simulink model "rotpentemplate"  (R2020b)
settings: Solver=ode45  StartTime=0.0  StopTime=30  RelTol=1e-3  EnableMultiTasking=on
values from neighbouring files (symbols this model uses):
  adingain = [adingain 1 1 1 1 1]    [hwinit.m]
  adinoffs = [adinoffs 0 0 0 0 0]    [hwinit.m]
  daoutgain = 1*[-6]    [hwinit.m]
  daoutoffs = -[-0.0025]    [hwinit.m]
undefined symbols (not defined in the file or in its folder): Discrete, h, Kd, Ld, R, sysd, Time
libraries: simulink x5, sharedTrackingLibrary x1, ctrlSharedLib x1
settings Model: Creator=rbabuska  LastModifiedBy=fballast
settings DataIOCC: LimitDataPoints=on  SaveFormat=Array  ReturnWorkspaceOutputs=off  SignalLoggingName=sigsOut
settings OptimizationCC: BooleanDataType=off  ExpressionDepthLimit=2147483647  InitFltsAndDblsToZero=on  LifeSpan=inf
settings DebuggingCC: SaveWithParameterizedLinksMsg=none  SignalResolutionControl=TryResolveAllWithWarning  MultiTaskDSMMsg=warning  MultiTaskCondExecSysMsg=none  AllowSymbolicDim=off  StateNameClashWarn=warning  SFUnexpectedBacktrackingDiag=warning  SFNoUnconditionalDefaultTransitionDiag=warning  SFExecutionAtInitializationDiag=none  ArithmeticOperatorsInVariantConditions=warning
settings HardwareCC: ProdBitPerPointer=32  ProdBitPerSizeT=32  ProdBitPerPtrDiffT=32  ProdLargestAtomicFloat=None  ProdIntDivRoundTo=Undefined  ProdEndianess=Unspecified  ProdWordSize=32  ProdHWDeviceType=32-bit Generic  TargetUnknown=on
settings ModelReferenceCC: PropagateSignalLabelsOutOfModel=off
settings SFSimCC: SimUseLocalCustomCode=off  CustomCodeUndefinedFunction=UseInterfaceOnly
settings RTWCC: RTWUseLocalCustomCode=off
settings CodeAppCC: StateflowObjectComments=on
settings GRTTargetCC: TargetFcnLib=ansi_tfl_tmw.mat  TargetLangStandard=C89/C90 (ANSI)  CombineOutputUpdateFcns=off  GRTInterface=on
settings ConfigComp: CovMetricSettings=dw  CovSaveCumulativeToWorkspaceVar=on  CovSaveSingleToWorkspaceVar=on  CovExternalEMLEnable=off

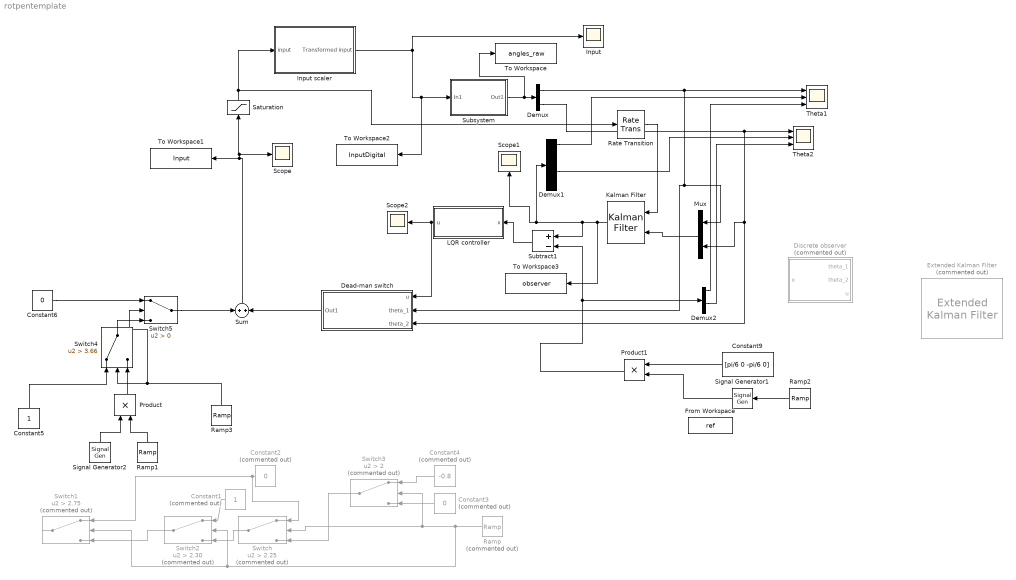
== system rotpentemplate ==
  Constant1 : Constant  Commented=on
  Constant2 : Constant  Commented=on  Value=0
  Constant3 : Constant  Commented=on  Value=0
  Constant4 : Constant  Commented=on  Value=-0.8
  Constant5 : Constant
  Constant6 : Constant  Value=0
  Constant9 : Constant  Value=[pi/6 0 -pi/6 0]
  Dead-man switch : Subsystem
  Demux : Demux  Outputs=2
  Demux1 : Demux
  Demux2 : Demux
  Discrete observer : Subsystem  Commented=on
  Extended Kalman Filter : sharedTrackingLibrary/Extended Kalman Filter  Commented=on  StateTransitionFcn=nonlin_state  HasStateTransitionJacobianFcn=off  HasAdditiveProcessNoise=Additive  ProcessNoise=Q  HasTimeVaryingProcessNoise=off  HasStateTransitionFcnExtraArgument=1  InitialState=[0;0;0;0]  InitialStateCovariance=1.0e-1  MeasurementFcn1=nonlin_meas  HasMeasurementJacobianFcn1=off  HasMeasurementEnablePort1=off  HasAdditiveMeasurementNoise1=Additive  MeasurementNoise1=R  HasTimeVaryingMeasurementNoise1=off  HasMeasurementFcnExtraArgument1=0  MeasurementFcn2=myMeasurementFcn  HasMeasurementJacobianFcn2=off  HasMeasurementEnablePort2=off  HasAdditiveMeasurementNoise2=Additive  MeasurementNoise2=1  HasTimeVaryingMeasurementNoise2=off  HasMeasurementFcnExtraArgument2=0  MeasurementFcn3=myMeasurementFcn  HasMeasurementJacobianFcn3=off  HasMeasurementEnablePort3=off  HasAdditiveMeasurementNoise3=Additive  MeasurementNoise3=1  HasTimeVaryingMeasurementNoise3=off  HasMeasurementFcnExtraArgument3=0  MeasurementFcn4=myMeasurementFcn  HasMeasurementJacobianFcn4=off  HasMeasurementEnablePort4=off  HasAdditiveMeasurementNoise4=Additive  MeasurementNoise4=1  HasTimeVaryingMeasurementNoise4=off  HasMeasurementFcnExtraArgument4=0  MeasurementFcn5=myMeasurementFcn  HasMeasurementJacobianFcn5=off  HasMeasurementEnablePort5=off  HasAdditiveMeasurementNoise5=Additive  MeasurementNoise5=1  HasTimeVaryingMeasurementNoise5=off  HasMeasurementFcnExtraArgument5=0  EnableMultirate=off  StateTransitionFcnSampleTime=1  MeasurementFcn1SampleTime=1  MeasurementFcn2SampleTime=1  MeasurementFcn3SampleTime=1  MeasurementFcn4SampleTime=1  MeasurementFcn5SampleTime=1  UseCurrentEstimator=on  OutputStateCovariance=off  DataType=double  SampleTime=0.01  NumberOfMeasurements=1
      settings: SourceProductBaseCode=CT,DR,TF,ID,LP,NV,AR,RO,RR,UV,VE
  From Workspace : FromWorkspace  VariableName=ref
  Input : Scope
  Input scaler : Subsystem
  Kalman Filter : ctrlSharedLib/Kalman Filter  TimeDomain=Discrete-Time  UseCurrentEstimator=on  ModelSource=LTI State-Space Variable  ModelSourceVariable=sysd  A=0.95  B=1  C=1  D=0  NumberOfStates=1  NumberOfInputs=1  NumberOfOutputs=1  InitialEstimateSource=Dialog  X0=0  P0=10  UseK=off  UseGH=off  NumberOfProcessNoiseInputs=1  G=eye(4)  TimeInvariantG=on  H=0  TimeInvariantH=on  Q=Q  TimeInvariantQ=on  R=R  TimeInvariantR=on  N=0  TimeInvariantN=on  AddInputPort=on  AddEnablePort=off  OutputEstimatedY=off  OutputP=off  Ts=-1
  LQR controller : Subsystem
  Mux : Mux  Inputs=2
  Product : Product
  Product1 : Product
  Ramp : simulink/Sources/Ramp  Commented=on  slope=1  start=0  InitialOutput=0
  Ramp1 : simulink/Sources/Ramp  slope=0.76  start=0.86  InitialOutput=0
  Ramp2 : simulink/Sources/Ramp  slope=1  start=3  InitialOutput=0
  Ramp3 : simulink/Sources/Ramp  slope=1  start=0  InitialOutput=0
  Rate Transition : RateTransition  OutPortSampleTime=h
  Saturation : Saturate  UpperLimit=1  LowerLimit=-1
  Scope : Scope
  Scope1 : Scope
  Scope2 : Scope
  Signal Generator1 : SignalGenerator  TimeSource=Use external signal  Amplitude=0  Frequency=0.1
  Signal Generator2 : SignalGenerator  Frequency=1.15
  Subsystem : Subsystem
      mask Display: disp('Rotational\nPendulum')
  Subtract1 : Sum  Inputs=+-
  Sum : Sum  Inputs=+|+
  Switch : Switch  Commented=on  Criteria=u2 > Threshold  Threshold=2.25
  Switch1 : Switch  Commented=on  Criteria=u2 > Threshold  Threshold=2.75
  Switch2 : Switch  Commented=on  Criteria=u2 > Threshold  Threshold=2.30
  Switch3 : Switch  Commented=on  Criteria=u2 > Threshold  Threshold=2
  Switch4 : Switch  Criteria=u2 > Threshold  Threshold=3.66
  Switch5 : Switch  Criteria=u2 > Threshold
  Theta1 : Scope  NumInputPorts=3
  Theta2 : Scope  NumInputPorts=3
  To Workspace : ToWorkspace  VariableName=angles_raw  SaveFormat=Timeseries  SampleTime=-1
  To Workspace1 : ToWorkspace  VariableName=Input  SaveFormat=Timeseries  SampleTime=-1
  To Workspace2 : ToWorkspace  VariableName=InputDigital  SaveFormat=Timeseries  SampleTime=-1
  To Workspace3 : ToWorkspace  VariableName=observer  SaveFormat=Timeseries  SampleTime=-1
  wires:
  Input scaler/1(Transformed input) -> To Workspace2/1, Subsystem/1(In1), Input/1
  Subsystem/1(Out1) -> To Workspace/1, Demux/1
  Demux/1 -> Theta1/1, Dead-man switch/2(theta_1), Mux/1
  Kalman Filter/1 -> To Workspace3/1, Subtract1/1, Scope1/1, Demux1/1
  Demux/2 -> Dead-man switch/3(theta_2), Mux/2, Theta2/1
  LQR controller/1(u) -> Scope2/1, Dead-man switch/1(u)
  Demux1/1 -> Theta1/2
  Demux1/3 -> Theta2/2
  Mux/1 -> Kalman Filter/2
  Rate Transition/1 -> Kalman Filter/1
  Subtract1/1 -> LQR controller/1(x)
  Demux2/1 -> Theta1/3
  Demux2/3 -> Theta2/3
  Ramp2/1 -> Signal Generator1/1
  Constant9/1 -> Product1/1
  Sum/1 -> To Workspace1/1, Scope/1, Saturation/1
  Switch3/1 -> Switch/3
  Ramp/1 -> Switch3/2, Switch/2, Switch2/2, Switch1/2
  Switch2/1 -> Switch1/3
  Constant2/1 -> Switch/1, Switch1/1
  Dead-man switch/1(Out1) -> Sum/2
  Constant1/1 -> Switch2/1
  Switch/1 -> Switch2/3
  Constant3/1 -> Switch3/3
  Constant4/1 -> Switch3/1
  Signal Generator2/1 -> Product/1
  Ramp1/1 -> Product/2
  Product/1 -> Switch4/3
  Constant5/1 -> Switch4/1
  Ramp3/1 -> Switch5/2, Switch4/2
  Switch5/1 -> Sum/1
  Constant6/1 -> Switch5/1
  Switch4/1 -> Switch5/3
  Product1/1 -> Subtract1/2, Demux2/1
  Saturation/1 -> Input scaler/1(input), Rate Transition/1
  Signal Generator1/1 -> Product1/2

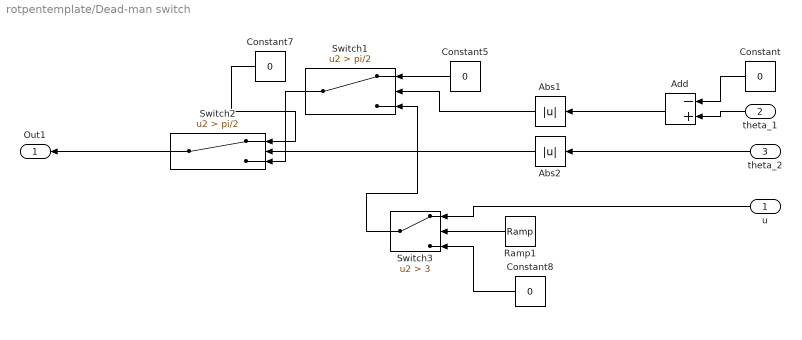
== system rotpentemplate/Dead-man switch ==
  u : Inport
  theta_1 : Inport  Port=2
  theta_2 : Inport  Port=3
  Abs1 : Abs
  Abs2 : Abs
  Add : Sum  Inputs=-+
  Constant{,5,7..8} (4 alike) : Constant  Value=0
  Ramp1 : simulink/Sources/Ramp  slope=1  start=0  InitialOutput=0
  Switch1 : Switch  Criteria=u2 > Threshold  Threshold=pi/2
  Switch2 : Switch  Criteria=u2 > Threshold  Threshold=pi/2
  Switch3 : Switch  Criteria=u2 > Threshold  Threshold=3
  Out1 : Outport
  wires:
  Switch3/1 -> Switch1/3
  Ramp1/1 -> Switch3/2
  Abs2/1 -> Switch2/2
  Abs1/1 -> Switch1/2
  Constant5/1 -> Switch1/1
  Constant7/1 -> Switch2/1
  Switch1/1 -> Switch2/3
  Constant8/1 -> Switch3/3
  theta_2/1 -> Abs2/1
  u/1 -> Switch3/1
  Switch2/1 -> Out1/1
  theta_1/1 -> Add/2
  Add/1 -> Abs1/1
  Constant/1 -> Add/1

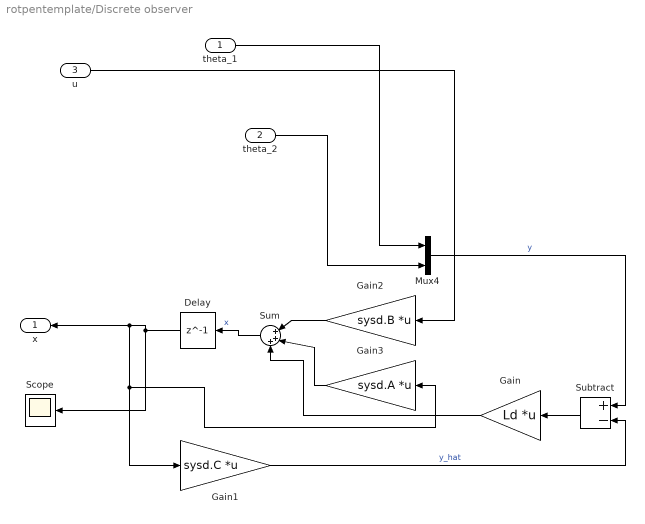
== system rotpentemplate/Discrete observer ==
  theta_1 : Inport
  theta_2 : Inport  Port=2
  u : Inport  Port=3
  Delay : Delay  DelayLength=1
  Gain : Gain  Gain=Ld  Multiplication=Matrix(K*u) (u vector)
  Gain1 : Gain  Gain=sysd.C  Multiplication=Matrix(K*u) (u vector)
  Gain2 : Gain  Gain=sysd.B  Multiplication=Matrix(K*u) (u vector)
  Gain3 : Gain  Gain=sysd.A  Multiplication=Matrix(K*u) (u vector)
  Mux4 : Mux  Inputs=2
  Scope : Scope
  Subtract : Sum  Inputs=+-
  Sum : Sum  Inputs=|+++
  x : Outport
  wires:
  Gain1/1 -> Subtract/2  "y_hat"
  theta_2/1 -> Mux4/2
  Subtract/1 -> Gain/1
  Gain/1 -> Sum/3
  Gain2/1 -> Sum/1
  Sum/1 -> Delay/1  "x"
  Mux4/1 -> Subtract/1  "y"
  Gain3/1 -> Sum/2
  u/1 -> Gain2/1
  theta_1/1 -> Mux4/1
  Delay/1 -> x/1, Gain3/1, Gain1/1, Scope/1

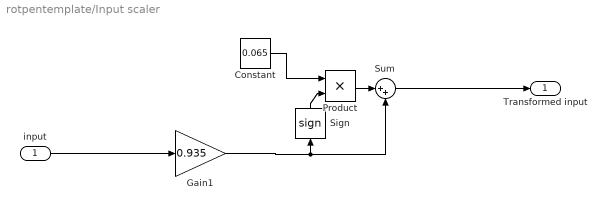
== system rotpentemplate/Input scaler ==
  input : Inport
  Constant : Constant  Value=0.065
  Gain1 : Gain  Gain=0.935
  Product : Product
  Sign : Signum
  Sum : Sum  Inputs=|++
  Transformed input : Outport
  wires:
  Gain1/1 -> Sum/2, Sign/1
  Constant/1 -> Product/1
  Sign/1 -> Product/2
  Sum/1 -> Transformed input/1
  Product/1 -> Sum/1
  input/1 -> Gain1/1

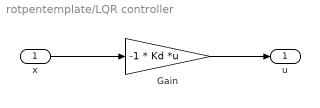
== system rotpentemplate/LQR controller ==
  x : Inport
  Gain : Gain  Gain=-1 * Kd  Multiplication=Matrix(K*u) (u vector)
  u : Outport
  wires:
  x/1 -> Gain/1
  Gain/1 -> u/1

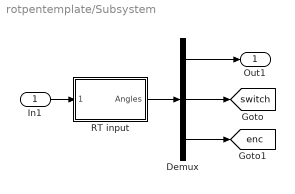
== system rotpentemplate/Subsystem ==
  In1 : Inport
  Demux : Demux  Outputs=[2 4 1]
  RT input : Subsystem  mask{Ts=h, channels=[6 7]}
      mask prompts: Ts "Sample time [s]:"; channels "Channels to read (e.g., [6 7])"
      mask init:
      | hwinit;
      | 
      | % initialize FPGA
      | fugihandle = fugiboard('Open', 'Pendulum1');
      | fugihandle.WatchdogTimeout = 0.5;
      | fugiboard('SetParams', fugihandle);
      | fugiboard('Write', fugihandle, 0, 0, 0, 0);  % dummy write to sync interface board
      | fugiboard('Write', fugihandle, 5, 1, 0, 0);  % reset position, activate relay
      | data = fugiboard('Read', fugihandle);        % get version info from FPGA
      | % model = bitshift(data(1), -5); 
      | % version = bitand(data(1), 31);
      | % disp(sprintf('FPGA setup %d, version %d', model, version)); % for the B&P it should say 1 1, or else there is a problem
      | fugiboard('Write', fugihandle, 0, 1, 0, 0);  % end reset
      | pause(0.1);                         % give relay some time to respond
      mask Display: disp('Rotational\nPendulum')
  Out1 : Outport
  tag scope: enc=global, switch=global
  wires:
  RT input/1(Angles) -> Demux/1
  Demux/1 -> Out1/1
  Demux/2 -> [switch]
  Demux/3 -> [enc]
  In1/1 -> RT input/1(Motors)

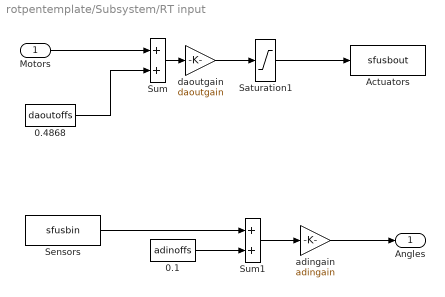
== system rotpentemplate/Subsystem/RT input ==
  Motors : Inport
  0.1 : Constant  Value=adinoffs
  0.4868 : Constant  Value=daoutoffs
  Actuators : S-Function  FunctionName=sfusbout  Parameters=Ts, fugihandle  SFunctionDeploymentMode=off  EnableBusSupport=off
  Saturation1 : Saturate  UpperLimit=10  LowerLimit=-10
  Sensors : S-Function  FunctionName=sfusbin  Parameters=Ts, fugihandle, channels  SFunctionDeploymentMode=off  EnableBusSupport=off
  Sum : Sum  InputSameDT=on  SaturateOnIntegerOverflow=on  OutDataTypeStr=Inherit: Same as first input
  Sum1 : Sum  InputSameDT=on  SaturateOnIntegerOverflow=on  OutDataTypeStr=Inherit: Same as first input
  adingain : Gain  Gain=adingain  SaturateOnIntegerOverflow=on  OutDataTypeStr=Inherit: Same as input  ParamDataTypeStr=Inherit: Same as input
  daoutgain : Gain  Gain=daoutgain  SaturateOnIntegerOverflow=on  OutDataTypeStr=Inherit: Same as input  ParamDataTypeStr=Inherit: Same as input
  Angles : Outport
  wires:
  Sum/1 -> daoutgain/1
  0.4868/1 -> Sum/2
  Motors/1 -> Sum/1
  Sum1/1 -> adingain/1
  0.1/1 -> Sum1/2
  adingain/1 -> Angles/1
  Saturation1/1 -> Actuators/1
  daoutgain/1 -> Saturation1/1
  Sensors/1 -> Sum1/1
